simulink model "CA1_model"  (R2023b)
settings: Solver=VariableStepAuto  StartTime=0.0  StopTime=2000  RelTol=1e-3
values from neighbouring files (symbols this model uses):
  a1 = 0.22    [CA1_param.m]    (also in CA1_param_change.m)
  a2 = 6.1    [CA1_param.m]    (also in CA1_param_change.m)
  b0 = -0.5    [CA1_param.m]    (also in CA1_param_change.m)
  b1 = -1    [CA1_param.m]    (also in CA1_param_change.m)
  Gamma = diag([10000*g,10000*g,1000*g,1000*g,1000*g])    [CA1_param.m]    (also in CA1_param_change.m)
  t1 = T(2)    [CA1_param.m]    (also in CA1_param_change.m)
  t2 = T(3)    [CA1_param.m]    (also in CA1_param_change.m)
  tau = 1/10    (= 0.1)    [CA1_param.m]    (also in CA1_param_change.m)
settings Model: Creator=99551  LastModifiedBy=99551
settings DebuggingCC: UnconnectedInputMsg=warning  UnconnectedOutputMsg=warning  UnconnectedLineMsg=warning
settings ModelReferenceCC: EnableRefExpFcnMdlSchedulingChecks=on
settings RTWCC: DLArmComputeVersion=19.05

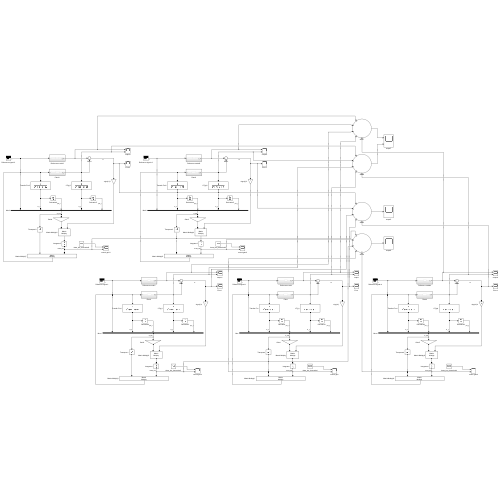
[thumbnail: Simulink's stored preview of the top-level diagram]
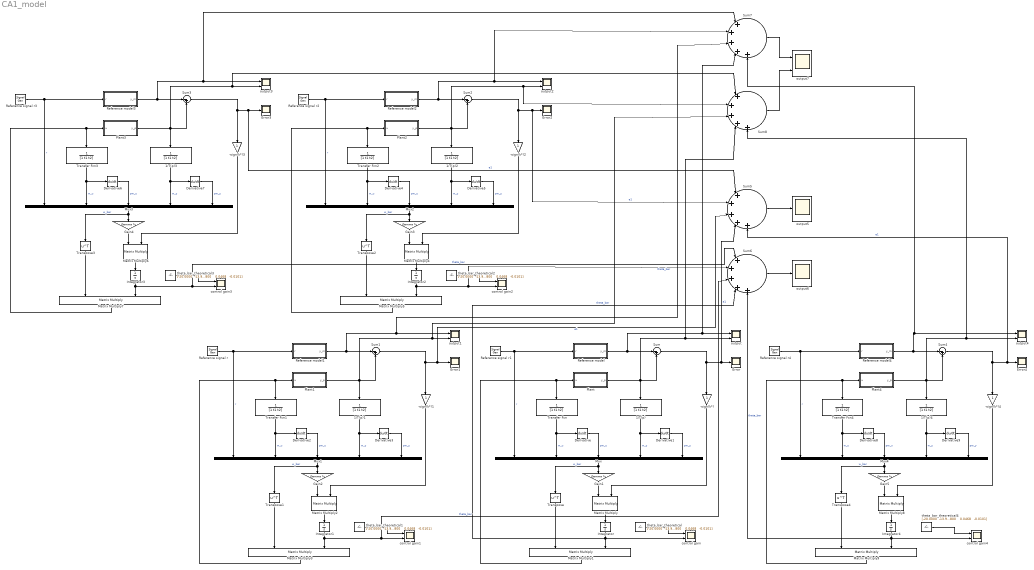
== system CA1_model ==
  -sign(k*){,1..4} (5 alike) : Gain
  1/T(p){,1..4} (5 alike) : TransferFcn  Denominator=[1 t1 t2]
  Derivative{,1..9} (10 alike) : Derivative
  Error{,1..4} (5 alike) : Scope
  Gain{1..5} (5 alike) : Gain  Gain=Gamma  Multiplication=Matrix(K*u)
  Integrator{,1..4} (5 alike) : Integrator
  Matrix Multiply{,1..9} (10 alike) : Product  Multiplication=Matrix(*)
  Mux{,1..4} (5 alike) : Mux  Inputs=5
  Plant : Subsystem
  Plant1 : Subsystem
  Plant2 : Subsystem
  Plant3 : Subsystem
  Plant4 : Subsystem
  Reference model : Subsystem
  Reference model1 : Subsystem
  Reference model2 : Subsystem
  Reference model3 : Subsystem
  Reference model4 : Subsystem
  Reference signal r : SignalGenerator  Amplitude=10  Frequency=0.0796
  Reference signal r1 : SignalGenerator  Amplitude=9  Frequency=0.0955
  Reference signal r2 : SignalGenerator  Amplitude=12  Frequency=0.0637
  Reference signal r3 : SignalGenerator  Amplitude=8  Frequency=0.0876
  Reference signal r4 : SignalGenerator  Amplitude=11  Frequency=0.0717
  Sum{,1..4} (5 alike) : Sum  Inputs=|-+
  Sum{5..8} (4 alike) : Sum  Inputs=|+++++
  Transfer Fcn{,1..4} (5 alike) : TransferFcn  Denominator=[1 t1 t2]
  Transpose{,1..4} (5 alike) : Math  Operator=transpose
  control gain{,1..4} (5 alike) : Scope  NumInputPorts=2
  output{,1..4,7} (6 alike) : Scope  NumInputPorts=2
  output5 : Scope
  output6 : Scope
  theta_bar_theoretical{,1..4} (5 alike) : Constant  Value="[-20.0000  -13.9037  -11.7800    0.0468   -0.0101]"
  wires:
  Reference model/1(y_m) -> Sum7/4, output/1, Sum/1
  Plant/1(y_p) -> Sum8/4, output/2, 1/T(p)/1, Sum/2
  Sum/1 -> Sum5/4, Error/1, -sign(k*)/1  "e1"
  Transfer Fcn/1 -> Mux/2, Derivative/1  "w_u"
  1/T(p)/1 -> Mux/4, Derivative1/1  "w_y"
  Derivative1/1 -> Mux/5  "pw_y"
  Derivative/1 -> Mux/3  "pw_u"
  Mux/1 -> Transpose/1, Gain1/1  "w_bar"
  Gain1/1 -> Matrix Multiply/1
  -sign(k*)/1 -> Matrix Multiply/2
  Matrix Multiply/1 -> Integrator/1
  Transpose/1 -> Matrix Multiply1/1
  Integrator/1 -> control gain/2, Sum6/4, Matrix Multiply1/2  "theta_bar"
  Matrix Multiply1/1 -> Transfer Fcn/1, Plant/1(u)
  theta_bar_theoretical/1 -> control gain/1
  Reference signal r1/1 -> Mux/1, Reference model/1(r)  "r"
  Derivative3/1 -> Mux1/5  "pw_y"
  Transfer Fcn1/1 -> Mux1/2, Derivative2/1  "w_u"
  Mux1/1 -> Transpose1/1, Gain2/1  "w_bar"
  Gain2/1 -> Matrix Multiply2/1
  Sum1/1 -> Sum5/3, Error1/1, -sign(k*)1/1  "e1"
  Reference model1/1(y_m) -> Sum7/3, output1/1, Sum1/1
  Matrix Multiply3/1 -> Transfer Fcn1/1, Plant1/1(u)
  theta_bar_theoretical1/1 -> control gain1/1
  Reference signal r/1 -> Mux1/1, Reference model1/1(r)  "r"
  1/T(p)1/1 -> Mux1/4, Derivative3/1  "w_y"
  Plant1/1(y_p) -> Sum8/3, output1/2, 1/T(p)1/1, Sum1/2
  Integrator1/1 -> Matrix Multiply3/2, Sum6/3, control gain1/2  "theta_bar"
  Transpose1/1 -> Matrix Multiply3/1
  Matrix Multiply2/1 -> Integrator1/1
  -sign(k*)1/1 -> Matrix Multiply2/2
  Derivative2/1 -> Mux1/3  "pw_u"
  Reference signal r3/1 -> Mux3/1, Reference model3/1(r)  "r"
  Plant3/1(y_p) -> Sum8/1, output3/2, 1/T(p)3/1, Sum3/2
  -sign(k*)3/1 -> Matrix Multiply6/2
  Matrix Multiply6/1 -> Integrator3/1
  Transpose3/1 -> Matrix Multiply7/1
  1/T(p)3/1 -> Mux3/4, Derivative7/1  "w_y"
  theta_bar_theoretical3/1 -> control gain3/1
  Sum3/1 -> Sum5/1, Error3/1, -sign(k*)3/1  "e1"
  Gain4/1 -> Matrix Multiply6/1
  Mux3/1 -> Transpose3/1, Gain4/1  "w_bar"
  Integrator3/1 -> Matrix Multiply7/2, Sum6/1, control gain3/2  "theta_bar"
  Derivative5/1 -> Mux2/5  "pw_y"
  Transfer Fcn2/1 -> Mux2/2, Derivative4/1  "w_u"
  Gain3/1 -> Matrix Multiply4/1
  Matrix Multiply7/1 -> Transfer Fcn3/1, Plant3/1(u)
  Mux2/1 -> Transpose2/1, Gain3/1  "w_bar"
  Reference model3/1(y_m) -> Sum7/1, output3/1, Sum3/1
  Transfer Fcn3/1 -> Mux3/2, Derivative6/1  "w_u"
  Sum2/1 -> Sum5/2, Error2/1, -sign(k*)2/1  "e1"
  Reference model2/1(y_m) -> Sum7/2, output2/1, Sum2/1
  Derivative7/1 -> Mux3/5  "pw_y"
  Matrix Multiply5/1 -> Transfer Fcn2/1, Plant2/1(u)
  theta_bar_theoretical2/1 -> control gain2/1
  Reference signal r2/1 -> Mux2/1, Reference model2/1(r)  "r"
  1/T(p)2/1 -> Mux2/4, Derivative5/1  "w_y"
  Plant2/1(y_p) -> Sum8/2, output2/2, 1/T(p)2/1, Sum2/2
  Integrator2/1 -> Matrix Multiply5/2, Sum6/2, control gain2/2  "theta_bar"
  Derivative6/1 -> Mux3/3  "pw_u"
  Transpose2/1 -> Matrix Multiply5/1
  Matrix Multiply4/1 -> Integrator2/1
  -sign(k*)2/1 -> Matrix Multiply4/2
  Derivative4/1 -> Mux2/3  "pw_u"
  Matrix Multiply9/1 -> Transfer Fcn4/1, Plant4/1(u)
  Sum4/1 -> Error4/1, Sum5/5, -sign(k*)4/1  "e1"
  Reference model4/1(y_m) -> output4/1, Sum7/5, Sum4/1
  Mux4/1 -> Transpose4/1, Gain5/1  "w_bar"
  Transfer Fcn4/1 -> Mux4/2, Derivative8/1  "w_u"
  Reference signal r4/1 -> Mux4/1, Reference model4/1(r)  "r"
  Gain5/1 -> Matrix Multiply8/1
  Derivative9/1 -> Mux4/5  "pw_y"
  -sign(k*)4/1 -> Matrix Multiply8/2
  Matrix Multiply8/1 -> Integrator4/1
  Derivative8/1 -> Mux4/3  "pw_u"
  Transpose4/1 -> Matrix Multiply9/1
  Integrator4/1 -> control gain4/2, Sum6/5, Matrix Multiply9/2  "theta_bar"
  Plant4/1(y_p) -> output4/2, Sum8/5, 1/T(p)4/1, Sum4/2
  1/T(p)4/1 -> Mux4/4, Derivative9/1  "w_y"
  theta_bar_theoretical4/1 -> control gain4/1
  Sum5/1 -> output5/1
  Sum6/1 -> output6/1
  Sum7/1 -> output7/1
  Sum8/1 -> output7/2

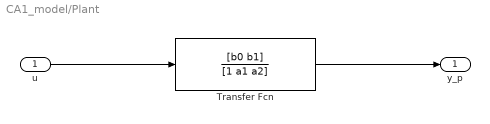
== system CA1_model/Plant ==
  u : Inport
  Transfer Fcn : TransferFcn  Numerator=[b0 b1]  Denominator=[1 a1 a2]
  y_p : Outport
  wires:
  u/1 -> Transfer Fcn/1
  Transfer Fcn/1 -> y_p/1

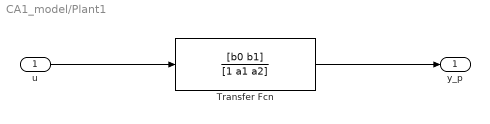
== system CA1_model/Plant1 ==
  u : Inport
  Transfer Fcn : TransferFcn  Numerator=[b0 b1]  Denominator=[1 a1 a2]
  y_p : Outport
  wires:
  u/1 -> Transfer Fcn/1
  Transfer Fcn/1 -> y_p/1

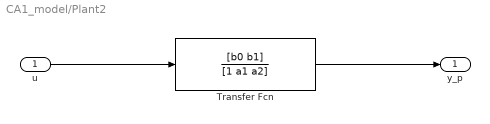
== system CA1_model/Plant2 ==
  u : Inport
  Transfer Fcn : TransferFcn  Numerator=[b0 b1]  Denominator=[1 a1 a2]
  y_p : Outport
  wires:
  u/1 -> Transfer Fcn/1
  Transfer Fcn/1 -> y_p/1

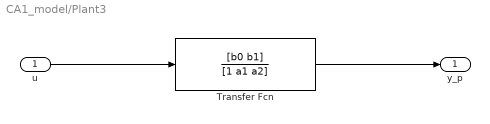
== system CA1_model/Plant3 ==
  u : Inport
  Transfer Fcn : TransferFcn  Numerator=[b0 b1]  Denominator=[1 a1 a2]
  y_p : Outport
  wires:
  u/1 -> Transfer Fcn/1
  Transfer Fcn/1 -> y_p/1

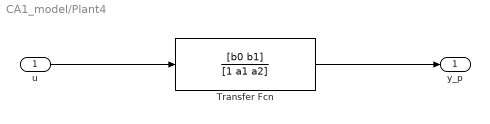
== system CA1_model/Plant4 ==
  u : Inport
  Transfer Fcn : TransferFcn  Numerator=[b0 b1]  Denominator=[1 a1 a2]
  y_p : Outport
  wires:
  u/1 -> Transfer Fcn/1
  Transfer Fcn/1 -> y_p/1

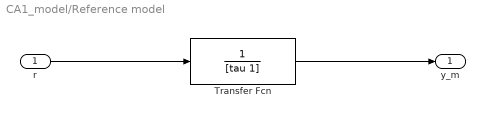
== system CA1_model/Reference model ==
  r : Inport
  Transfer Fcn : TransferFcn  Denominator=[tau 1]
  y_m : Outport
  wires:
  Transfer Fcn/1 -> y_m/1
  r/1 -> Transfer Fcn/1

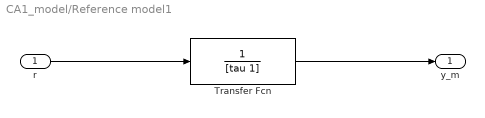
== system CA1_model/Reference model1 ==
  r : Inport
  Transfer Fcn : TransferFcn  Denominator=[tau 1]
  y_m : Outport
  wires:
  Transfer Fcn/1 -> y_m/1
  r/1 -> Transfer Fcn/1

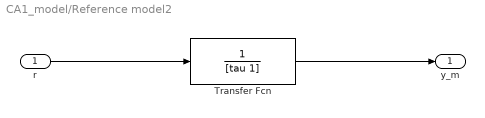
== system CA1_model/Reference model2 ==
  r : Inport
  Transfer Fcn : TransferFcn  Denominator=[tau 1]
  y_m : Outport
  wires:
  Transfer Fcn/1 -> y_m/1
  r/1 -> Transfer Fcn/1

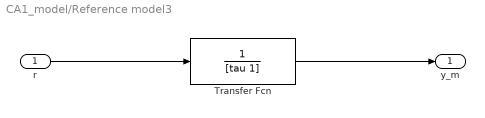
== system CA1_model/Reference model3 ==
  r : Inport
  Transfer Fcn : TransferFcn  Denominator=[tau 1]
  y_m : Outport
  wires:
  Transfer Fcn/1 -> y_m/1
  r/1 -> Transfer Fcn/1

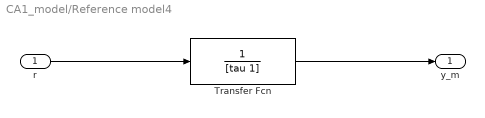
== system CA1_model/Reference model4 ==
  r : Inport
  Transfer Fcn : TransferFcn  Denominator=[tau 1]
  y_m : Outport
  wires:
  Transfer Fcn/1 -> y_m/1
  r/1 -> Transfer Fcn/1
